simulink model "N3_TE0722A5"  (R2014a)
settings: Solver=ode45  StartTime=0.0  StopTime=1e-4  RelTol=1e-3
PreLoadFcn:
  | fpgaclk=1/32.768e6
  | SerialData=[1,zeros(1,11),1,0,0,1]
  | load ../window
  | win=win'   %Go back to using flatter and wider windowed sync function
  | %load ../hanning    %use Hahn window
  | 
  | load ../PREemphasis   %For pre-empasis and deemphasis FIRs
  | 
  | LUT3=xls2LUT2('../IQI_Qdemod.xls')
  | load ../FIRiq2
  | % xls2LUT
  | 
  | GetProgFiles
  | 
  | PinAssignments    %Get Pin references for TE0722
  | 
  | 
  | 
  | 
  | 
  | %LCD
  | LCDdata=[LCD_D7,LCD_D6,LCD_D5,LCD_D4,LCD_D3,LCD_D2,LCD_D1,LCD_D0] %Note MSB...LSB!
  | LCDctrl=[LCD_E,LCD_RW,LCD_RS];
  | 
  | %for RS232 on pins 3 and 5 of USBB
  | 
  | %BT chip connections for WT12
  | 
  | RX_BT=RXD
  | TX_BT=TXD
  | 
  | RST_BB=RES
  | 
  | %PCMC=PCMC
  | %PCMS=PCMS
  | %PCMI=PCMI
  | %PCMO=PCMO
  | 
  | %Aliases:
  | SRDBT=PCMI
  | STDBT=PCMO
  | SCLK_BT=PCMC
  | SFS_BT=PCMS
  | 
  | %ADC control
  | 
  | %SDOA=SDOA
  | %SDOB=SDOB
  | %SCK=SCK
  | CONV=Csbar
  | CAL=Cal
  | 
  | ADC_G=[ADC_G3,ADC_G2,ADC_G1,ADC_G0]
  | %PD settings hard coded now
  | 
  | %%%%%%
  | TX_LOW=TX_Low
  | 
  | %Leds
  | %Defined inPinassignments
  | 
  | 
  | 
  | %TouchPads
  | %Defined in Pinassignments
  | 
  | 
  | 'Got to end of pre-load OK'
StartFcn:
  | fpgaclk=1/32.768e6
  | SerialData=[1,zeros(1,11),1,0,0,1]
values from neighbouring files (symbols this model uses):
  ADC_G0 = {'P10'}    [PinAssignments.m]
  ADC_G1 = {'P11'}    [PinAssignments.m]
  ADC_G2 = {'N14'}    [PinAssignments.m]
  ADC_G3 = {'M11'}    [PinAssignments.m]
  Cal = {'L12'}    [PinAssignments.m]
  Csbar = {'M12'}    [PinAssignments.m]
  LCD_D0 = {'J13'}    [PinAssignments.m]
  LCD_D1 = {'J14'}    [PinAssignments.m]
  LCD_D2 = {'F15'}    [PinAssignments.m]
  LCD_D3 = {'H14'}    [PinAssignments.m]
  LCD_D4 = {'G12'}    [PinAssignments.m]
  LCD_D5 = {'L15'}    [PinAssignments.m]
  LCD_D6 = {'M14'}    [PinAssignments.m]
  LCD_D7 = {'K15'}    [PinAssignments.m]
  PCMC = {'H11'}    [PinAssignments.m]
  PCMI = {'H12'}    [PinAssignments.m]
  PCMO = {'N13'}    [PinAssignments.m]
  PCMS = {'M10'}    [PinAssignments.m]
  RES = {'G11'}    [PinAssignments.m]
  RXD = {'H13'}    [PinAssignments.m]
  TX_Low = {'P15'}    [PinAssignments.m]
  TXD = {'P13'}    [PinAssignments.m]
undefined symbols (not defined in the file or in its folder): FIRRX, FIRTX
libraries: xbsIndex_r4 x1100, MyFunctions x42
(part 1 of 9)
settings Model: Creator=Graham  LastModifiedBy=gnaylor
settings DataIOCC: SignalLoggingSaveFormat=ModelDataLogs  SignalLoggingName=sigsOut
settings OptimizationCC: ExpressionDepthLimit=2147483647  InitFltsAndDblsToZero=on
settings DebuggingCC: SaveWithParameterizedLinksMsg=none  UnderspecifiedInitializationDetection=Classic  SignalResolutionControl=TryResolveAllWithWarning  SolverPrmCheckMsg=none  MultiTaskDSMMsg=warning  MultiTaskCondExecSysMsg=none  InvalidFcnCallConnMsg=warning  FcnCallInpInsideContextMsg=EnableAllAsWarning  StateNameClashWarn=warning
settings HardwareCC: TargetUnknown=on
settings RTWCC: IncludeERTFirstTime=on
settings GRTTargetCC: TargetFcnLib=ansi_tfl_tmw.mat  ModelReferenceCompliant=off  CombineOutputUpdateFcns=off  MatFileLogging=off  GRTInterface=on

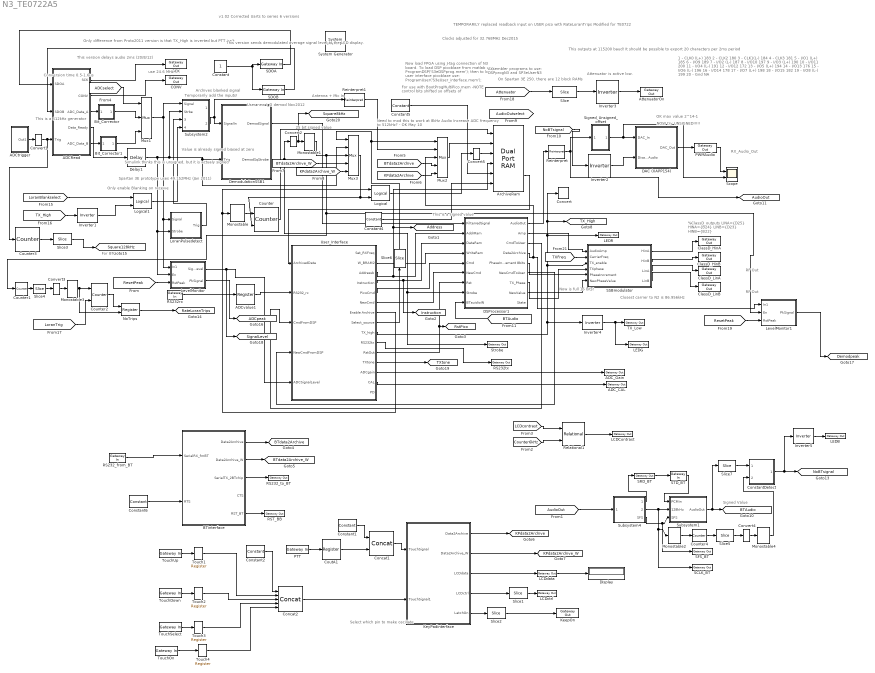
== system N3_TE0722A5 ==
  note: v1.02 Corrected Uarts to series 6 versions
  note: OK max value 2^14-1
  note: This outputs at 115200 baud! It should be possible to export 20 characters per 2ms period
  note: 1 - CLK0 (L+)	183	2 - CLK2	180
      | 3 - CLK1(L-)	184	4 - CLK3	181
      | 5 - I/O1 (L+)	185	6 - I/O9	189
      | 7 - I/O2 (L-)	187	8 - I/O10	197
      | 9 - I/O3 (L+)	190	10 - I/O11	200
      | 11 - I/O4 (L-)	191	12 - I/O12	172
      | 13 - I/O5 (L+)	194	14 - I/O13	176
      | 15 - I/O6 (L-)	196	16 - I/O14	178
      | 17 - I/O7 (L+)	198	18 - I/O15	182
      | 19 - I/O8 (L-)	199	20 - Gnd	NA
  note: This is a 512kHz generator
  note: use 24.6 MHz
  note: Spartan 3E prototype uses 49.152MHz (Jan 2011)
  note: Conversion time 0.5-1.6us
  note: RX_Audio_Out
  note: RF Out
  note: Antenna + Mic In
  note: Now load FPGA using J-tag connection
      | of N3 board.
      | To load DSP picoblaze from matlab use:
      | ProgramDSP('S3eDSPprog.mem');
      | then to load user interface picoblaze use:
      | ProgramUser('S3eUser_interface.mem');
  note: Assembler programs to use:
      | DSPprogN3 and
      | SP3eUserN3
  note: Value is already signed biased at zero
  note: This is a signed value
  note: For use with BootProgMultiPico.mem
      | -NOTE control bits shifted so offsets of
  note: Need to mod this to work at 8kHz Audio
      | Increase ADC frequency to 512kHz? - OK May 10
  note: Closest carrier to N2 is 86.956kHz
  note: 25 bit signed value
  note: Simulink thinks this is unsigned, but it is actualy signed
  note: Clocks adjusted for 32.768MHz Dec2015
  note: Select which pin to make oscillate
  note: %ClassD_outputs
      | LINA={D25}
      | HINA={B24}
      | LINB={D23}
      | HINB={B22}
  note: RF Out
  note: On Spartan 3E 250, there are 12 block RAMs
  note: NOW try UNSIGNED!!!!!
  note: Temporarily add the inputs!
  note: Now is
      | full 16 bits!
  note: Only difference from Proto2011 version is that TX_High is inverted but PTT isn't
  note: Archives blanked signal
  note: Only enable Blanking on receive
  note: This version delays audio 2ms (20/8/12)
  note: Uses new I_Q demod Nov2012
  note: TEMPORARILY replaced readback input on USER pico with RateLoranTrips
      | Modified for TE0722
  note: Signed Value
  note: For BT
  note: Attenuator is active low.
  note: This version sends demodulated average signal level to the LCD display.
  " System Generator" : xbsIndex_r4/ System Generator  Tag=genX  xilinxfamily=zynq  part=xc7z010  speed=-1  package=clg225  synthesis_tool=XST  clock_wrapper=Clock Enables  directory=C:/SysgenOutput/TE0722GVA5  proj_type=Project Navigator  Synth_file=XST Defaults  Impl_file=ISE Defaults  testbench=off  simulink_period=fpgaclk  sysclk_period=30  dcm_input_clock_period=100  incr_netlist=off  trim_vbits=Everywhere in SubSystem  dbl_ovrd=According to Block Masks  core_generation=According to Block Masks  run_coregen=off  deprecated_control=off  eval_field=0  block_type=sysgen
      settings: block_version=8.2.02
  ADCRead : Subsystem
  ADC_CAL : xbsIndex_r4/Gateway Out  inherit_from_input=off  hdl_port=on  rows=1  columns=1  UseAsDAC=off  DACChannel='1'  interface=None  automatic_assignment=on  address_offset=hex2dec('00')  intf_description=''  timing_constraint=None  locs_specified=on  LOCs=CAL  io_standard={'LVCMOS33'}  block_type=gatewayout
      settings: block_version=VER_STRING_GOES_HERE
  ADC_Gain : xbsIndex_r4/Gateway Out  inherit_from_input=off  hdl_port=on  rows=1  columns=1  UseAsDAC=off  DACChannel='1'  interface=None  automatic_assignment=on  address_offset=hex2dec('00')  intf_description=''  timing_constraint=None  locs_specified=on  LOCs=ADC_G  io_standard={'LVCMOS','LVCMOS','LVCMOS','LVCMOS'}  block_type=gatewayout
      settings: block_version=VER_STRING_GOES_HERE
  ADCtrigger : Subsystem
  ADCvalue1 : xbsIndex_r4/Register  init=0  rst=off  en=off  dbl_ovrd=off  block_type=register
      settings: xl_area=[0, 0, 0, 0, 0, 0, 0]  block_version=VER_STRING_GOES_HERE
  ArchiveRam : xbsIndex_r4/Dual Port RAM  depth=1024*4  initVector=zeros(1,4096)  distributed_mem=Block RAM  init_a=0  init_b=0  rst_a=off  rst_b=off  en_a=off  en_b=off  latency=1  write_mode_A=Read After Write  write_mode_B=Read After Write  optimize=Area  dbl_ovrd=off  block_type=dpram
      settings: block_version=8.2.02
  AttenuatorOn : xbsIndex_r4/Gateway Out  inherit_from_input=off  hdl_port=on  rows=1  columns=1  UseAsDAC=off  DACChannel='1'  interface=None  automatic_assignment=on  address_offset=hex2dec('00')  intf_description=''  timing_constraint=None  locs_specified=on  LOCs=Atten  io_standard={'LVCMOS33'}  block_type=gatewayout
      settings: xl_area=[0, 0, 0, 0, 0, 0, 0]  block_version=VER_STRING_GOES_HERE
  BTinterface : Subsystem
  Bit_Corrector : Subsystem  TreatAsAtomicUnit=on
  Bit_Corrector1 : Subsystem  TreatAsAtomicUnit=on
  CONV : xbsIndex_r4/Gateway Out  inherit_from_input=off  hdl_port=on  rows=1  columns=1  UseAsDAC=off  DACChannel='1'  interface=None  automatic_assignment=on  address_offset=hex2dec('00')  intf_description=''  timing_constraint=None  locs_specified=on  LOCs=CONV  io_standard={'LVCMOS33'}  block_type=gatewayout
      settings: xl_area=[0, 0, 0, 0, 0, 0, 0]  block_version=VER_STRING_GOES_HERE
  ClassD_HinA : xbsIndex_r4/Gateway Out  inherit_from_input=off  hdl_port=on  rows=1  columns=1  UseAsDAC=off  DACChannel='1'  interface=None  automatic_assignment=on  address_offset=hex2dec('00')  intf_description=''  timing_constraint=None  locs_specified=on  LOCs=HINA  io_standard={'LVCMOS33'}  block_type=gatewayout
      settings: xl_area=[0, 0, 0, 0, 0, 0, 0]  block_version=VER_STRING_GOES_HERE
  ClassD_HinB : xbsIndex_r4/Gateway Out  inherit_from_input=off  hdl_port=on  rows=1  columns=1  UseAsDAC=off  DACChannel='1'  interface=None  automatic_assignment=on  address_offset=hex2dec('00')  intf_description=''  timing_constraint=None  locs_specified=on  LOCs=HINB  io_standard={'LVCMOS33'}  block_type=gatewayout
      settings: xl_area=[0, 0, 0, 0, 0, 0, 0]  block_version=VER_STRING_GOES_HERE
  ClassD_LinA : xbsIndex_r4/Gateway Out  inherit_from_input=off  hdl_port=on  rows=1  columns=1  UseAsDAC=off  DACChannel='1'  interface=None  automatic_assignment=on  address_offset=hex2dec('00')  intf_description=''  timing_constraint=None  locs_specified=on  LOCs=LINA  io_standard={'LVCMOS33'}  block_type=gatewayout
      settings: xl_area=[0, 0, 0, 0, 0, 0, 0]  block_version=VER_STRING_GOES_HERE
  ClassD_LinB : xbsIndex_r4/Gateway Out  inherit_from_input=off  hdl_port=on  rows=1  columns=1  UseAsDAC=off  DACChannel='1'  interface=None  automatic_assignment=on  address_offset=hex2dec('00')  intf_description=''  timing_constraint=None  locs_specified=on  LOCs=LINB  io_standard={'LVCMOS33'}  block_type=gatewayout
      settings: xl_area=[0, 0, 0, 0, 0, 0, 0]  block_version=VER_STRING_GOES_HERE
  Concat1 : xbsIndex_r4/Concat  num_inputs=2  dbl_ovrd=off  block_type=concat
      settings: block_version=12.2
  Concat2 : xbsIndex_r4/Concat  num_inputs=5  dbl_ovrd=off  block_type=concat
      settings: block_version=12.2
  Constant : Constant
  Constant1 : xbsIndex_r4/Constant  const=0  gui_display_data_type=Fixed-point  arith_type=Unsigned  n_bits=7  bin_pt=0  preci_type=Single  exp_width=8  frac_width=24  explicit_period=on  period=fpgaclk  equ=P=C  opselect=C  inp2=PCIN>>17  opr=+  inp1=P  carry=CIN  dbl_ovrd=off  block_type=constant
      settings: block_version=VER_STRING_GOES_HERE
  Constant2 : xbsIndex_r4/Constant  const=0  gui_display_data_type=Fixed-point  arith_type=Unsigned  n_bits=4  bin_pt=0  preci_type=Single  exp_width=8  frac_width=24  explicit_period=on  period=fpgaclk  equ=P=C  opselect=C  inp2=PCIN>>17  opr=+  inp1=P  carry=CIN  dbl_ovrd=off  block_type=constant
      settings: block_version=VER_STRING_GOES_HERE
  Constant4 : xbsIndex_r4/Constant  const=0  gui_display_data_type=Boolean  arith_type=Boolean  n_bits=1  bin_pt=0  preci_type=Single  exp_width=8  frac_width=24  explicit_period=on  period=fpgaclk  equ=P=C  opselect=C  inp2=PCIN>>17  opr=+  inp1=P  carry=CIN  dbl_ovrd=off  block_type=constant
      settings: block_version=VER_STRING_GOES_HERE
  Constant5 : xbsIndex_r4/Constant  const=0  gui_display_data_type=Fixed-point  arith_type=Unsigned  n_bits=16  bin_pt=0  preci_type=Single  exp_width=8  frac_width=24  explicit_period=on  period=fpgaclk  equ=P=C  opselect=C  inp2=PCIN>>17  opr=+  inp1=P  carry=CIN  dbl_ovrd=off  block_type=constant
      settings: block_version=VER_STRING_GOES_HERE
  Constant6 : xbsIndex_r4/Constant  const=1  gui_display_data_type=Fixed-point  arith_type=Unsigned  n_bits=1  bin_pt=0  preci_type=Single  exp_width=8  frac_width=24  explicit_period=on  period=fpgaclk  equ=P=C  opselect=C  inp2=PCIN>>17  opr=+  inp1=P  carry=CIN  dbl_ovrd=off  block_type=constant
      settings: block_version=VER_STRING_GOES_HERE
  ConstantDetect : Subsystem
  Convert : xbsIndex_r4/Convert  gui_display_data_type=Fixed-point  arith_type=Boolean  n_bits=16  bin_pt=14  float_type=Single  exp_bits=8  fraction_bits=24  quantization=Truncate  overflow=Wrap  en=off  latency=0  pipeline=off  dbl_ovrd=off  block_type=convert
      settings: block_version=8.2.02
  Convert1 : xbsIndex_r4/Convert  gui_display_data_type=Fixed-point  arith_type=Boolean  n_bits=8  bin_pt=6  float_type=Single  exp_bits=8  fraction_bits=24  quantization=Truncate  overflow=Wrap  en=off  latency=0  pipeline=off  dbl_ovrd=off  block_type=convert
      settings: xl_area=[0 0 0 0 0 0 0]  block_version=VER_STRING_GOES_HERE
  Convert2 : xbsIndex_r4/Convert  gui_display_data_type=Boolean  arith_type=Boolean  n_bits=16  bin_pt=0  float_type=Single  exp_bits=8  fraction_bits=24  quantization=Truncate  overflow=Wrap  en=off  latency=0  pipeline=off  dbl_ovrd=off  block_type=convert
      settings: xl_area=[0, 0, 0, 0, 0, 0, 0]  block_version=VER_STRING_GOES_HERE
  Convert3 : xbsIndex_r4/Convert  gui_display_data_type=Fixed-point  arith_type=Boolean  n_bits=16  bin_pt=14  float_type=Single  exp_bits=8  fraction_bits=24  quantization=Truncate  overflow=Wrap  en=off  latency=0  pipeline=off  dbl_ovrd=off  block_type=convert
      settings: block_version=8.2.02
  Convert4 : xbsIndex_r4/Convert  gui_display_data_type=Fixed-point  arith_type=Boolean  n_bits=8  bin_pt=6  float_type=Single  exp_bits=8  fraction_bits=24  quantization=Truncate  overflow=Wrap  en=off  latency=0  pipeline=off  dbl_ovrd=off  block_type=convert
      settings: xl_area=[0 0 0 0 0 0 0]  block_version=VER_STRING_GOES_HERE
  Convert5 : xbsIndex_r4/Convert  gui_display_data_type=Fixed-point  arith_type=Boolean  n_bits=16  bin_pt=14  float_type=Single  exp_bits=8  fraction_bits=24  quantization=Truncate  overflow=Wrap  en=off  latency=0  pipeline=off  dbl_ovrd=off  block_type=convert
      settings: block_version=8.2.02
  Counter : xbsIndex_r4/Counter  cnt_type=Free Running  cnt_to=Inf  operation=Up  start_count=0  cnt_by_val=1  arith_type=Unsigned  n_bits=12  bin_pt=0  load_pin=off  rst=on  en=on  explicit_period=off  period=1  use_behavioral_HDL=off  implementation=Fabric  use_rpm=off  dbl_ovrd=off  block_type=counter
      settings: block_version=8.2.02
  Counter1 : xbsIndex_r4/Counter  cnt_type=Free Running  cnt_to=Inf  operation=Up  start_count=0  cnt_by_val=1  arith_type=Unsigned  n_bits=13  bin_pt=0  load_pin=off  rst=off  en=on  explicit_period=off  period=1  use_behavioral_HDL=off  implementation=Fabric  use_rpm=off  dbl_ovrd=off  block_type=counter
      settings: block_version=8.2.02
  Counter2 : xbsIndex_r4/Counter  cnt_type=Free Running  cnt_to=Inf  operation=Up  start_count=0  cnt_by_val=1  arith_type=Unsigned  n_bits=8  bin_pt=0  load_pin=off  rst=on  en=on  explicit_period=off  period=1  use_behavioral_HDL=off  implementation=Fabric  use_rpm=off  dbl_ovrd=off  block_type=counter
      settings: block_version=8.2.02
  Counter3 : xbsIndex_r4/Counter  cnt_type=Free Running  cnt_to=Inf  operation=Up  start_count=0  cnt_by_val=1  arith_type=Unsigned  n_bits=2  bin_pt=0  load_pin=off  rst=off  en=on  explicit_period=on  period=fpgaclk  use_behavioral_HDL=off  implementation=Fabric  dbl_ovrd=off  block_type=counter
      settings: block_version=12.2
  Counter4 : xbsIndex_r4/Counter  cnt_type=Free Running  cnt_to=Inf  operation=Up  start_count=0  cnt_by_val=1  arith_type=Unsigned  n_bits=4  bin_pt=0  load_pin=off  rst=off  en=on  explicit_period=on  period=fpgaclk  use_behavioral_HDL=off  implementation=Fabric  dbl_ovrd=off  block_type=counter
      settings: block_version=12.2
  CoutA1 : xbsIndex_r4/Register  init=0  rst=off  en=off  dbl_ovrd=off  block_type=register
      settings: xl_area=[0, 0, 0, 0, 0, 0, 0]  block_version=VER_STRING_GOES_HERE
  DAC (XAPP154) : Subsystem
  DSProcessor1 : Subsystem
  Delay1 : xbsIndex_r4/Delay  rst=off  infoeditControl=Selection of Reset will increase slice count due to use of real FFs and instead of SRLs  en=off  latency=2  reg_retiming=off  dbl_ovrd=off  block_type=delay
      settings: xl_area=[1 1 0 0 0 0 0]  block_version=VER_STRING_GOES_HERE
  DemodulationSSB1 : Subsystem
  Display : Display
  Inverter{1..5} (5 alike) : xbsIndex_r4/Inverter  en=off  latency=0  dbl_ovrd=off  block_type=inv
      settings: block_version=12.2
  KeepOn : xbsIndex_r4/Gateway Out  inherit_from_input=off  hdl_port=on  rows=1  columns=1  UseAsDAC=off  DACChannel='1'  interface=None  automatic_assignment=on  address_offset=hex2dec('00')  intf_description=''  timing_constraint=None  locs_specified=on  LOCs=Keep_On  io_standard={'LVCMOS33'}  block_type=gatewayout
      settings: xl_area=[0, 0, 0, 0, 0, 0, 0]  block_version=VER_STRING_GOES_HERE
  KeyPadinterface : Subsystem
  LCDContrast : xbsIndex_r4/Gateway Out  inherit_from_input=off  hdl_port=on  rows=1  columns=1  UseAsDAC=off  DACChannel='1'  interface=None  automatic_assignment=on  address_offset=hex2dec('00')  intf_description=''  timing_constraint=None  locs_specified=on  LOCs=LCD_V0  io_standard={'LVCMOS33'}  block_type=gatewayout
      settings: block_version=VER_STRING_GOES_HERE
  LCDctrl : xbsIndex_r4/Gateway Out  inherit_from_input=off  hdl_port=on  rows=1  columns=1  UseAsDAC=off  DACChannel='1'  interface=None  automatic_assignment=on  address_offset=hex2dec('00')  intf_description=''  timing_constraint=None  locs_specified=on  LOCs=LCDctrl  io_standard={'LVCMOS33','LVCMOS33','LVCMOS33'}  block_type=gatewayout
      settings: block_version=VER_STRING_GOES_HERE
  LCDdata : xbsIndex_r4/Gateway Out  inherit_from_input=off  hdl_port=on  rows=1  columns=1  UseAsDAC=off  DACChannel='1'  interface=None  automatic_assignment=on  address_offset=hex2dec('00')  intf_description=''  timing_constraint=None  locs_specified=on  LOCs=LCDdata  io_standard={'LVCMOS33','LVCMOS33','LVCMOS33','LVCMOS33','LVCMOS33','LVCMOS33','LVCMOS33','LVCMOS33'}  block_type=gatewayout
      settings: block_version=VER_STRING_GOES_HERE
  LEDB : xbsIndex_r4/Gateway Out  inherit_from_input=off  hdl_port=on  rows=1  columns=1  UseAsDAC=off  DACChannel='1'  interface=None  automatic_assignment=on  address_offset=hex2dec('00')  intf_description=''  timing_constraint=None  locs_specified=on  LOCs=RGB_B  io_standard={'LVCMOS33'}  block_type=gatewayout
      settings: block_version=VER_STRING_GOES_HERE
  LEDG : xbsIndex_r4/Gateway Out  inherit_from_input=off  hdl_port=on  rows=1  columns=1  UseAsDAC=off  DACChannel='1'  interface=None  automatic_assignment=on  address_offset=hex2dec('00')  intf_description=''  timing_constraint=None  locs_specified=on  LOCs=RGB_G  io_standard={'LVCMOS33'}  block_type=gatewayout
      settings: block_version=VER_STRING_GOES_HERE
  LEDR : xbsIndex_r4/Gateway Out  inherit_from_input=off  hdl_port=on  rows=1  columns=1  UseAsDAC=off  DACChannel='1'  interface=None  automatic_assignment=on  address_offset=hex2dec('00')  intf_description=''  timing_constraint=None  locs_specified=on  LOCs=RGB_R  io_standard={'LVCMOS33'}  block_type=gatewayout
      settings: block_version=VER_STRING_GOES_HERE
  LevelMonitor : Subsystem
  LevelMonitor1 : Subsystem
  Logical : xbsIndex_r4/Logical  logical_function=AND  inputs=2  en=off  latency=2  precision=Full  arith_type=Unsigned  n_bits=16  bin_pt=0  align_bp=on  dbl_ovrd=off  block_type=logical
      settings: block_version=8.2.02
  Logical1 : xbsIndex_r4/Logical  logical_function=AND  inputs=2  en=off  latency=1  precision=Full  arith_type=Unsigned  n_bits=16  bin_pt=0  align_bp=on  dbl_ovrd=off  block_type=logical
      settings: block_version=8.2.02
  LoranPulsedetect : Subsystem
  Monostable : MyFunctions/Monostable
  Monostable1 : MyFunctions/Monostable
      link override Delay1: en=off  latency=1  dbl_ovrd=off  reg_retiming=off
      link override Delay1: infoedit=Hardware notes: A delay line is a chain, each link of which is an SRL16 followed by a flip-flop.  xl_area=[0, 0, 0, 0, 0, 0, 0]
  Monostable2 : MyFunctions/Monostable
      link override Delay1: xl_area=[1 1 0 0 0 0 0]
      link override Inverter: xl_area=[0 0 0 0 0 0 0]
      link override Logical: xl_area=[1 0 0 1 0 0 0]
  Monostable3 : MyFunctions/Monostable
      link override Delay1: en=off  latency=1  dbl_ovrd=off  reg_retiming=off
      link override Delay1: infoedit=Hardware notes: A delay line is a chain, each link of which is an SRL16 followed by a flip-flop.  xl_area=[0, 0, 0, 0, 0, 0, 0]
  Monostable4 : MyFunctions/Monostable
      link override Delay1: xl_area=[1 1 0 0 0 0 0]
      link override Inverter: xl_area=[0 0 0 0 0 0 0]
      link override Logical: xl_area=[1 0 0 1 0 0 0]
  Mux1 : xbsIndex_r4/Mux  inputs=2  en=off  latency=1  precision=Full  arith_type=Unsigned  n_bits=16  bin_pt=14  quantization=Truncate  overflow=Wrap  dbl_ovrd=off  block_type=mux
      settings: block_version=VER_STRING_GOES_HERE
  Mux2 : xbsIndex_r4/Mux  inputs=4  en=off  latency=1  precision=Full  arith_type=Unsigned  n_bits=16  bin_pt=14  quantization=Truncate  overflow=Wrap  dbl_ovrd=off  block_type=mux
      settings: block_version=VER_STRING_GOES_HERE
  Mux3 : xbsIndex_r4/Mux  inputs=4  en=off  latency=1  precision=Full  arith_type=Unsigned  n_bits=16  bin_pt=14  quantization=Truncate  overflow=Wrap  dbl_ovrd=off  block_type=mux
      settings: block_version=VER_STRING_GOES_HERE
  NoTrips : xbsIndex_r4/Register  init=0  rst=off  en=on  dbl_ovrd=off  block_type=register
      settings: xl_area=[0, 0, 0, 0, 0, 0, 0]  block_version=VER_STRING_GOES_HERE
  PTT : xbsIndex_r4/Gateway In  gui_display_data_type=Fixed-point  arith_type=Unsigned  n_bits=1  bin_pt=0  preci_type=Single  exp_width=8  frac_width=24  rows=1  columns=1  quantization="Round  (unbiased: +/- Inf)"  overflow=Saturate  period=fpgaclk  UseAsADC=off  ADCChannel='1'  interface=None  automatic_assignment=on  address_offset=hex2dec('00')  intf_description=''  timing_constraint=None  locs_specified=on  LOCs=PTT  io_standard={'LVCMOS33'}  inherit_from_input=off  hdl_port=on  dbl_ovrd=off  block_type=gatewayin
      settings: xl_area=[0, 0, 0, 0, 0, 0, 0]  block_version=VER_STRING_GOES_HERE
  PWMAudio : xbsIndex_r4/Gateway Out  inherit_from_input=off  hdl_port=on  rows=1  columns=1  UseAsDAC=off  DACChannel='1'  interface=None  automatic_assignment=on  address_offset=hex2dec('00')  intf_description=''  timing_constraint=None  locs_specified=on  LOCs=PWMAudio  io_standard={'LVCMOS33'}  block_type=gatewayout
      settings: xl_area=[0, 0, 0, 0, 0, 0, 0]  block_version=VER_STRING_GOES_HERE
  RS232_from_BT : xbsIndex_r4/Gateway In  gui_display_data_type=Fixed-point  arith_type=Unsigned  n_bits=1  bin_pt=0  preci_type=Single  exp_width=8  frac_width=24  rows=1  columns=1  quantization="Round  (unbiased: +/- Inf)"  overflow=Saturate  period=fpgaclk  UseAsADC=off  ADCChannel='1'  interface=None  automatic_assignment=on  address_offset=hex2dec('00')  intf_description=''  timing_constraint=None  locs_specified=on  LOCs=TX_BT  io_standard={'LVCMOS33'}  inherit_from_input=off  hdl_port=on  dbl_ovrd=off  block_type=gatewayin
      settings: block_version=VER_STRING_GOES_HERE
  RS232_to_BT : xbsIndex_r4/Gateway Out  inherit_from_input=off  hdl_port=on  rows=1  columns=1  UseAsDAC=off  DACChannel='1'  interface=None  automatic_assignment=on  address_offset=hex2dec('00')  intf_description=''  timing_constraint=None  locs_specified=on  LOCs=RX_BT  io_standard={'LVCMOS33'}  block_type=gatewayout
      settings: block_version=VER_STRING_GOES_HERE
  RS232rx : xbsIndex_r4/Gateway In  gui_display_data_type=Fixed-point  arith_type=Unsigned  n_bits=1  bin_pt=0  preci_type=Single  exp_width=8  frac_width=24  rows=1  columns=1  quantization="Round  (unbiased: +/- Inf)"  overflow=Saturate  period=fpgaclk  UseAsADC=off  ADCChannel='1'  interface=None  automatic_assignment=on  address_offset=hex2dec('00')  intf_description=''  timing_constraint=None  locs_specified=on  LOCs=RS232rx  io_standard={'LVCMOS33'}  inherit_from_input=off  hdl_port=on  dbl_ovrd=off  block_type=gatewayin
      settings: block_version=VER_STRING_GOES_HERE
  RS232tx : xbsIndex_r4/Gateway Out  inherit_from_input=off  hdl_port=on  rows=1  columns=1  UseAsDAC=off  DACChannel='1'  interface=None  automatic_assignment=on  address_offset=hex2dec('00')  intf_description=''  timing_constraint=None  locs_specified=on  LOCs=RS232tx  io_standard={'LVCMOS33'}  block_type=gatewayout
      settings: block_version=VER_STRING_GOES_HERE
  RST_BB : xbsIndex_r4/Gateway Out  inherit_from_input=off  hdl_port=on  rows=1  columns=1  UseAsDAC=off  DACChannel='1'  interface=None  automatic_assignment=on  address_offset=hex2dec('00')  intf_description=''  timing_constraint=None  locs_specified=on  LOCs=RST_BB  io_standard={'LVCMOS'}  block_type=gatewayout
      settings: block_version=VER_STRING_GOES_HERE
  Reinterpret : xbsIndex_r4/Reinterpret  force_arith_type=on  arith_type="Signed  (2's comp)"  force_bin_pt=on  bin_pt=0  block_type=cast
      settings: block_version=VER_STRING_GOES_HERE
  Reinterpret1 : xbsIndex_r4/Reinterpret  force_arith_type=on  arith_type=Unsigned  force_bin_pt=on  bin_pt=0  block_type=reinterpret
      settings: infoedit="Changes signal type without altering the binary representation.   You can changed the signal between signed and unsigned, and relocate the binary point.<br><br>Hardware notes: In hardware this block costs nothing.<br><br>Example:  Suppose the input is 6 bits wide, signed, with 2 fractional bits, and the output is forced to unsigned with 0 fractional bits.  Then an input of -2.0 (1110.00 in binary 2's complement) becomes an output of 56 (111000 in binary)."  block_version=8.2.02
  Relational1 : xbsIndex_r4/Relational  mode=a>b  op_type=Bool  en=off  latency=1  dbl_ovrd=off  block_type=relational
      settings: block_version=10.1
  SCK : xbsIndex_r4/Gateway Out  inherit_from_input=off  hdl_port=on  rows=1  columns=1  UseAsDAC=off  DACChannel='1'  interface=None  automatic_assignment=on  address_offset=hex2dec('00')  intf_description=''  timing_constraint=None  locs_specified=on  LOCs=SCK  io_standard={'LVCMOS33'}  block_type=gatewayout
      settings: xl_area=[0, 0, 0, 0, 0, 0, 0]  block_version=VER_STRING_GOES_HERE
  SCLK_BT : xbsIndex_r4/Gateway Out  inherit_from_input=off  hdl_port=on  rows=1  columns=1  UseAsDAC=off  DACChannel='1'  interface=None  automatic_assignment=on  address_offset=hex2dec('00')  intf_description=''  timing_constraint=None  locs_specified=on  LOCs=SCLK_BT  io_standard={'LVCMOS33'}  block_type=gatewayout
      settings: block_version=VER_STRING_GOES_HERE
  SDOA : xbsIndex_r4/Gateway In  gui_display_data_type=Fixed-point  arith_type=Unsigned  n_bits=1  bin_pt=0  preci_type=Single  exp_width=8  frac_width=24  rows=1  columns=1  quantization="Round  (unbiased: +/- Inf)"  overflow=Saturate  period=fpgaclk  UseAsADC=off  ADCChannel='1'  interface=None  automatic_assignment=on  address_offset=hex2dec('00')  intf_description=''  timing_constraint=None  locs_specified=on  LOCs=SDOA  io_standard={'LVCMOS33'}  inherit_from_input=off  hdl_port=on  dbl_ovrd=off  block_type=gatewayin
      settings: xl_area=[0, 0, 0, 0, 0, 0, 0]  block_version=VER_STRING_GOES_HERE
  SDOB : xbsIndex_r4/Gateway In  gui_display_data_type=Fixed-point  arith_type=Unsigned  n_bits=1  bin_pt=0  preci_type=Single  exp_width=8  frac_width=24  rows=1  columns=1  quantization="Round  (unbiased: +/- Inf)"  overflow=Saturate  period=fpgaclk  UseAsADC=off  ADCChannel='1'  interface=None  automatic_assignment=on  address_offset=hex2dec('00')  intf_description=''  timing_constraint=None  locs_specified=on  LOCs=SDOB  io_standard={'LVCMOS33'}  inherit_from_input=off  hdl_port=on  dbl_ovrd=off  block_type=gatewayin
      settings: xl_area=[0, 0, 0, 0, 0, 0, 0]  block_version=VER_STRING_GOES_HERE
  SFS_BT : xbsIndex_r4/Gateway Out  inherit_from_input=off  hdl_port=on  rows=1  columns=1  UseAsDAC=off  DACChannel='1'  interface=None  automatic_assignment=on  address_offset=hex2dec('00')  intf_description=''  timing_constraint=None  locs_specified=on  LOCs=SFS_BT  io_standard={'LVCMOS33'}  block_type=gatewayout
      settings: block_version=VER_STRING_GOES_HERE
  SRD_BT : xbsIndex_r4/Gateway Out  inherit_from_input=off  hdl_port=on  rows=1  columns=1  UseAsDAC=off  DACChannel='1'  interface=None  automatic_assignment=on  address_offset=hex2dec('00')  intf_description=''  timing_constraint=None  locs_specified=on  LOCs=SRDBT  io_standard={'LVCMOS33'}  block_type=gatewayout
      settings: block_version=VER_STRING_GOES_HERE
  "SSBmodulator " : Subsystem
  STD_BT : xbsIndex_r4/Gateway In  gui_display_data_type=Fixed-point  arith_type=Unsigned  n_bits=1  bin_pt=0  preci_type=Single  exp_width=8  frac_width=24  rows=1  columns=1  quantization="Round  (unbiased: +/- Inf)"  overflow=Saturate  period=fpgaclk  UseAsADC=off  ADCChannel='1'  interface=None  automatic_assignment=on  address_offset=hex2dec('00')  intf_description=''  timing_constraint=None  locs_specified=on  LOCs=STDBT  io_standard={'LVCMOS33'}  inherit_from_input=off  hdl_port=on  dbl_ovrd=off  block_type=gatewayin
      settings: block_version=VER_STRING_GOES_HERE
  Scope : Scope  NumInputPorts=2
      settings: YMin=0~7782.4  YMax=1~8601.6
  Signed_Unsigned_offset : Subsystem
  Slice : xbsIndex_r4/Slice  nbits=1  boolean_output=off  mode=Lower Bit Location + Width  bit1=0  base1=MSB of Input  bit0=0  base0=LSB of Input  dbl_ovrd=off  block_type=slice
  Slice1 : xbsIndex_r4/Slice  nbits=3  boolean_output=off  mode=Lower Bit Location + Width  bit1=0  base1=MSB of Input  bit0=0  base0=LSB of Input  dbl_ovrd=off  block_type=slice
      settings: block_version=VER_STRING_GOES_HERE
  Slice2 : xbsIndex_r4/Slice  nbits=1  boolean_output=off  mode=Lower Bit Location + Width  bit1=0  base1=MSB of Input  bit0=0  base0=LSB of Input  dbl_ovrd=off  block_type=slice
      settings: block_version=VER_STRING_GOES_HERE
  Slice3 : xbsIndex_r4/Slice  nbits=1  boolean_output=off  mode=Upper Bit Location + Width  bit1=0  base1=MSB of Input  bit0=0  base0=LSB of Input  dbl_ovrd=off  block_type=slice
      settings: block_version=VER_STRING_GOES_HERE
  Slice4 : xbsIndex_r4/Slice  nbits=1  boolean_output=off  mode=Upper Bit Location + Width  bit1=0  base1=MSB of Input  bit0=0  base0=LSB of Input  dbl_ovrd=off  block_type=slice
      settings: block_version=VER_STRING_GOES_HERE
  Slice5 : xbsIndex_r4/Slice  nbits=1  boolean_output=off  mode=Upper Bit Location + Width  bit1=0  base1=MSB of Input  bit0=0  base0=LSB of Input  dbl_ovrd=off  block_type=slice
      settings: block_version=VER_STRING_GOES_HERE
  Slice6 : xbsIndex_r4/Slice  nbits=2  boolean_output=off  mode=Lower Bit Location + Width  bit1=0  base1=MSB of Input  bit0=0  base0=LSB of Input  dbl_ovrd=off  block_type=slice
      settings: block_version=VER_STRING_GOES_HERE
  Slice7 : xbsIndex_r4/Slice  nbits=8  boolean_output=off  mode=Lower Bit Location + Width  bit1=0  base1=MSB of Input  bit0=0  base0=LSB of Input  dbl_ovrd=off  block_type=slice
      settings: block_version=VER_STRING_GOES_HERE
  Strobe : xbsIndex_r4/Gateway Out  inherit_from_input=off  hdl_port=on  rows=1  columns=1  UseAsDAC=off  DACChannel='1'  interface=None  automatic_assignment=on  address_offset=hex2dec('00')  intf_description=''  timing_constraint=None  locs_specified=on  LOCs=Strobe  io_standard={'LVCMOS33'}  block_type=gatewayout
      settings: block_version=VER_STRING_GOES_HERE
  Subsystem1 : Subsystem
  Subsystem2 : Subsystem
  Subsystem4 : Subsystem
  TX_Low : xbsIndex_r4/Gateway Out  inherit_from_input=off  hdl_port=on  rows=1  columns=1  UseAsDAC=off  DACChannel='1'  interface=None  automatic_assignment=on  address_offset=hex2dec('00')  intf_description=''  timing_constraint=None  locs_specified=on  LOCs=TX_LOW  io_standard={'LVCMOS33'}  block_type=gatewayout
      settings: block_version=VER_STRING_GOES_HERE
  Touch{1..4} (4 alike) : xbsIndex_r4/Register  init=0  rst=off  en=off  dbl_ovrd=off  block_type=register
      settings: xl_area=[0, 0, 0, 0, 0, 0, 0]  block_version=VER_STRING_GOES_HERE
  TouchDown : xbsIndex_r4/Gateway In  gui_display_data_type=Fixed-point  arith_type=Unsigned  n_bits=1  bin_pt=0  preci_type=Single  exp_width=8  frac_width=24  rows=1  columns=1  quantization="Round  (unbiased: +/- Inf)"  overflow=Saturate  period=fpgaclk  UseAsADC=off  ADCChannel='1'  interface=None  automatic_assignment=on  address_offset=hex2dec('00')  intf_description=''  timing_constraint=None  locs_specified=on  LOCs=TouchDown  io_standard={'LVCMOS'}  inherit_from_input=off  hdl_port=on  dbl_ovrd=off  block_type=gatewayin
      settings: xl_area=[0, 0, 0, 0, 0, 0, 0]  block_version=VER_STRING_GOES_HERE
  TouchOn : xbsIndex_r4/Gateway In  gui_display_data_type=Fixed-point  arith_type=Unsigned  n_bits=1  bin_pt=0  preci_type=Single  exp_width=8  frac_width=24  rows=1  columns=1  quantization="Round  (unbiased: +/- Inf)"  overflow=Saturate  period=fpgaclk  UseAsADC=off  ADCChannel='1'  interface=None  automatic_assignment=on  address_offset=hex2dec('00')  intf_description=''  timing_constraint=None  locs_specified=on  LOCs=TouchOn  io_standard={'LVCMOS'}  inherit_from_input=off  hdl_port=on  dbl_ovrd=off  block_type=gatewayin
      settings: xl_area=[0, 0, 0, 0, 0, 0, 0]  block_version=VER_STRING_GOES_HERE
  TouchSelect : xbsIndex_r4/Gateway In  gui_display_data_type=Fixed-point  arith_type=Unsigned  n_bits=1  bin_pt=0  preci_type=Single  exp_width=8  frac_width=24  rows=1  columns=1  quantization="Round  (unbiased: +/- Inf)"  overflow=Saturate  period=fpgaclk  UseAsADC=off  ADCChannel='1'  interface=None  automatic_assignment=on  address_offset=hex2dec('00')  intf_description=''  timing_constraint=None  locs_specified=on  LOCs=TouchSelect  io_standard={'LVCMOS'}  inherit_from_input=off  hdl_port=on  dbl_ovrd=off  block_type=gatewayin
      settings: xl_area=[0, 0, 0, 0, 0, 0, 0]  block_version=VER_STRING_GOES_HERE
  TouchUp : xbsIndex_r4/Gateway In  gui_display_data_type=Fixed-point  arith_type=Unsigned  n_bits=1  bin_pt=0  preci_type=Single  exp_width=8  frac_width=24  rows=1  columns=1  quantization="Round  (unbiased: +/- Inf)"  overflow=Saturate  period=fpgaclk  UseAsADC=off  ADCChannel='1'  interface=None  automatic_assignment=on  address_offset=hex2dec('00')  intf_description=''  timing_constraint=None  locs_specified=on  LOCs=TouchUp  io_standard={'LVCMOS33'}  inherit_from_input=off  hdl_port=on  dbl_ovrd=off  block_type=gatewayin
      settings: xl_area=[0, 0, 0, 0, 0, 0, 0]  block_version=VER_STRING_GOES_HERE
  User_Interface : Subsystem
  tag scope: ADCpeak=global, Address=global, AudioOut=global, BTAudio=global, BTdata2Archive=global, BTdata2Archive_W=global, Demodpeak=global, Instruction=global, KPdata2Archive=global, KPdata2Archive_W=global, NoBTsignal=global, RateLoranTrips=global, RstPico=global, SignalLevel=global, Square128kHz=global, Square8kHz=global, TX_High=global, TXtone=global
  wires:
  ADCRead/1(SCK) -> SCK/1
  SDOA/1 -> ADCRead/1(SDOA)
  Constant/1 -> SDOA/1, SDOB/1
  ADCRead/2(CONV) -> CONV/1
  PWMAudio/1 -> Scope/1
  DAC (XAPP154)/1(DAC_Out) -> PWMAudio/1
  ADCtrigger/1(Out1) -> Convert1/1
  Convert1/1 -> ADCRead/3(Trig), Counter3/1
  ADCRead/4(Data_Ready) -> Delay1/1
  Reinterpret/1 -> [AudioOut], Signed_Unsigned_offset/1(In1)
  Subsystem2/2(CleanedUp) -> Reinterpret1/1, DemodulationSSB1/1(SignalIn)
  DemodulationSSB1/1(DemodSignal) -> DSProcessor1/1(FilterredSignal)
  User_Interface/2(W_BRAM2) -> DSProcessor1/4(WriteRam)
  User_Interface/3(Addressb) -> ArchiveRam/4, [Address], DSProcessor1/2(AddrRam)
  User_Interface/4(Instruction) -> [Instruction], DSProcessor1/3(DataRam)
  Counter/1 -> ArchiveRam/1
  ArchiveRam/2 -> User_Interface/1(ArchivedData)
  Mux2/1 -> ArchiveRam/2
  Monostable/1 -> Counter/1
  User_Interface/7(Enable Archive) -> Monostable/1, Logical/1
  User_Interface/8(Select_source) -> Slice6/1
  DSProcessor1/4(Data2Archive) -> LevelMonitor1/1(In1), Mux2/3
  DemodulationSSB1/2(DemodSqStrobe) -> Convert2/1, DSProcessor1/8(Strobe), Strobe/1
  Mux3/1 -> Counter/2, Logical/2
  Logical/1 -> Convert5/1
  DSProcessor1/1(AudioOut) -> Reinterpret/1
  User_Interface/5(PicoCmd) -> DSProcessor1/5(Cmd)
  DSProcessor1/2(Amp) -> "SSBmodulator "/1(AudioAmp)
  "SSBmodulator "/1(HinA) -> ClassD_HinA/1
  "SSBmodulator "/2(HinB) -> ClassD_HinB/1
  User_Interface/11(RstOut) -> DSProcessor1/7(Rst), [RstPico]
  User_Interface/6(NewCmd) -> DSProcessor1/6(NewCmd)
  Constant4/1 -> ArchiveRam/6
  Constant5/1 -> ArchiveRam/5
  Monostable1/1 -> Mux3/3, LevelMonitor1/2(En), Counter1/1
  Convert2/1 -> Monostable1/1, [Square8kHz]
  DSProcessor1/3(CmdToUser) -> User_Interface/3(CmdFromDSP)
  DSProcessor1/6(NewCmdToUser) -> User_Interface/4(NewCmdFromDSP)
  User_Interface/13(ADCgain) -> ADC_Gain/1
  Relational1/1 -> LCDContrast/1
  [Counter6kHz] -> Relational1/2
  [LCDcontrast] -> Relational1/1
  User_Interface/14(CAL) -> ADC_CAL/1
  SDOB/1 -> ADCRead/2(SDOB)
  ADCRead/3(ADC_Data_A) -> Bit_Corrector/1(In1)
  ADCRead/5(ADC_Data_B) -> Bit_Corrector1/1(In1)
  Delay1/1 -> Mux3/2, DemodulationSSB1/2(Trig), Subsystem2/2(Strbe), LoranPulsedetect/2(Strobe), LevelMonitor/2(En)
  KeyPadinterface/4(LCDctrl) -> Slice1/1
  LCDdata/1 -> Display/1
  Slice1/1 -> LCDctrl/1
  KeyPadinterface/3(LCDdata) -> LCDdata/1
  BTinterface/5(RST_BT) -> RST_BB/1
  BTinterface/1(Data2Archive) -> [BTdata2Archive]
  BTinterface/2(Data2Archive_W) -> [BTdata2Archive_W]
  KeyPadinterface/2(Data2Archive_W) -> [KPdata2Archive_W]
  KeyPadinterface/1(Data2Archive) -> [KPdata2Archive]
  [BTdata2Archive_W] -> Mux3/4
  [KPdata2Archive_W] -> Mux3/5
  [BTdata2Archive] -> Mux2/4
  [KPdata2Archive] -> Mux2/5
  Slice6/1 -> Mux2/1, Mux3/1
  Convert5/1 -> ArchiveRam/3
  Mux1/1 -> LevelMonitor/1(In1), LoranPulsedetect/1(Signal), Subsystem2/1(Signal)
  KeyPadinterface/5(LatchOn) -> Slice2/1
  TouchUp/1 -> Touch1/1
  TouchDown/1 -> Touch2/1
  TouchSelect/1 -> Touch3/1
  [AudioOut] -> Subsystem4/1(AudioIn)
  [BTAudio] -> DSProcessor1/9(BTauidioIN)
  [ADCselect] -> Mux1/1
  "SSBmodulator "/3(LinA) -> ClassD_LinA/1
  "SSBmodulator "/4(LinB) -> ClassD_LinB/1
  Constant6/1 -> BTinterface/2(RTS)
  RS232_from_BT/1 -> BTinterface/1(SerialRX_fmBT)
  RS232rx/1 -> ADCvalue1/1
  ADCvalue1/1 -> User_Interface/2(RS232_rx)
  Constant1/1 -> Concat1/1
  CoutA1/1 -> Concat1/2
  Concat1/1 -> KeyPadinterface/1(TouchSignal)
  BTinterface/3(SerialTX_2BTchip) -> RS232_to_BT/1
  Bit_Corrector/1(Out1) -> Mux1/2
  Bit_Corrector1/1(Out1) -> Mux1/3
  Reinterpret1/1 -> Mux2/2
  LevelMonitor/1(SignalLevel) -> [SignalLevel], User_Interface/5(ADCSignalLevel)
  DSProcessor1/7(TX_Phase) -> "SSBmodulator "/4(TXphase)
  PTT/1 -> CoutA1/1
  LoranPulsedetect/1(Trig) -> Subsystem2/3(LoranPulseTrig)
  [TX_High] -> Inverter1/1
  [LoranBlankselect] -> Logical1/1
  Inverter1/1 -> Logical1/2
  Logical1/1 -> Subsystem2/4(EnableGating)
  DSProcessor1/5(PhaseIncrement 8bits) -> "SSBmodulator "/5(PhaseIncrement)
  DSProcessor1/8(NewValue) -> "SSBmodulator "/6(NewPhaseValue)
  Counter1/1 -> Slice4/1
  Slice4/1 -> Convert3/1
  Monostable3/1 -> Counter2/1, NoTrips/2
  Counter2/1 -> NoTrips/1
  NoTrips/1 -> [RateLoranTrips]
  [LoranTrig] -> Counter2/2
  Convert3/1 -> Monostable3/1
  [NoBTsignal] -> Inverter2/1
  Subsystem4/3(SFS) -> Subsystem1/3(SFS), SFS_BT/1
  Subsystem4/2(128kHz) -> Subsystem1/2(128kHz), Monostable2/1, SCLK_BT/1
  Subsystem4/1(PCMout) -> SRD_BT/1
  STD_BT/1 -> Subsystem1/1(PCMin)
  SRD_BT/1 -> STD_BT/1
  Subsystem1/1(AudioOut) -> [BTAudio], Slice7/1
  ConstantDetect/1(IsConstant) -> Inverter5/1, [NoBTsignal]
  Slice7/1 -> ConstantDetect/1(Signal)
  Counter3/1 -> Slice3/1
  Slice3/1 -> [Square128kHz]
  Slice5/1 -> Convert4/1
  Convert4/1 -> Monostable4/1
  Monostable2/1 -> Counter4/1
  Monostable4/1 -> ConstantDetect/2(Strobe)
  Counter4/1 -> Slice5/1
  Constant2/1 -> Concat2/1
  Touch1/1 -> Concat2/2
  Touch2/1 -> Concat2/3
  Touch3/1 -> Concat2/4
  Concat2/1 -> KeyPadinterface/2(TouchSignal1)
  TouchOn/1 -> Touch4/1
  Touch4/1 -> Concat2/5
  [Attenuator] -> Slice/1
  Slice/1 -> Inverter3/1
  Inverter3/1 -> AttenuatorOn/1
  Slice2/1 -> KeepOn/1
  LevelMonitor/2(PkSignal) -> [ADCpeak]
  [ResetPeak] -> LevelMonitor/3(RstPeak)
  LevelMonitor1/1(PkSignal) -> [Demodpeak]
  [ResetPeak] -> LevelMonitor1/3(RstPeak)
  User_Interface/9(TX_high) -> Convert/1, [TX_High], LEDR/1, "SSBmodulator "/3(TX_enable), Inverter4/1
  [TXFreq] -> "SSBmodulator "/2(CarrierFreq)
  User_Interface/12(TXtone) -> [TXtone]
  Inverter2/1 -> DAC (XAPP154)/2(Disable_Audio)
  Signed_Unsigned_offset/1(Out1) -> Scope/2, DAC (XAPP154)/1(DAC_In)
  Inverter4/1 -> LEDG/1, TX_Low/1
  User_Interface/10(RS232tx) -> RS232tx/1
  Inverter5/1 -> LEDB/1

== system N3_TE0722A5/ADCRead ==
  note: 27 slices using Serial to parallel block
  note: 32 slices with Async triggering
  note: Trig on rising edge
  SDOA : Inport
  SDOB : Inport  Port=2
  Trig : Inport  Port=3
  Subsystem1 : Subsystem
  SCK : Outport
  CONV : Outport  Port=2
  ADC_Data_A : Outport  Port=3
  Data_Ready : Outport  Port=4
  ADC_Data_B : Outport  Port=5
  wires:
  SDOA/1 -> Subsystem1/1(SDOA)
  Subsystem1/2(Conv) -> CONV/1
  Subsystem1/1(ADCValueA) -> ADC_Data_A/1
  Subsystem1/3(SCK) -> SCK/1
  Subsystem1/4(DataReady) -> Data_Ready/1
  Trig/1 -> Subsystem1/2(Trig)
  SDOB/1 -> Subsystem1/3(SDOB)
  Subsystem1/5(ADCValueB) -> ADC_Data_B/1

== system N3_TE0722A5/ADCtrigger ==
  note: 214748 to generate 512kHz with 40MHz clock
      | 174762 for 49.152MHz
      | 262143 for 32.768MHz
  Accumulator1 : xbsIndex_r4/Accumulator  operation=Add  n_bits=24  overflow=Wrap  scale=1  rst=off  hasbypass=off  infoeditControl=reset for floating point data type must be asserted for a minimum of 2 cycles  en=off  latency=0  msb_inp=100  msb=100  lsb=-100  use_behavioral_HDL=on  implementation=Fabric  dbl_ovrd=off  block_type=accum
      settings: xl_area=[8 16 0 16 0 0 0]  block_version=VER_STRING_GOES_HERE
  Constant1 : xbsIndex_r4/Constant  const=262143  gui_display_data_type=Fixed-point  arith_type=Unsigned  n_bits=20  bin_pt=0  preci_type=Single  exp_width=8  frac_width=24  explicit_period=on  period=fpgaclk  equ=P=C  opselect=C  inp2=PCIN>>17  opr=+  inp1=P  carry=CIN  dbl_ovrd=off  block_type=constant
      settings: block_version=VER_STRING_GOES_HERE
  Monostable1 : MyFunctions/Monostable
  Slice2 : xbsIndex_r4/Slice  nbits=1  boolean_output=off  mode=Upper Bit Location + Width  bit1=0  base1=MSB of Input  bit0=0  base0=LSB of Input  dbl_ovrd=off  block_type=slice
      settings: infoedit="Extracts a given range of bits from each input sample and presents it at the output.  The output type is ordinarily unsigned with binary point at zero, but can be Boolean when the slice is one bit wide.<P><P>Hardware notes: In hardware this block costs nothing."  block_version=VER_STRING_GOES_HERE
  Out1 : Outport
  wires:
  Constant1/1 -> Accumulator1/1
  Accumulator1/1 -> Slice2/1
  Slice2/1 -> Monostable1/1
  Monostable1/1 -> Out1/1
